simulink model "SERIAL_TRANSMIT_LCD"  (R2021b)
settings: Solver=FixedStepAuto  StartTime=0.0  StopTime=inf  RelTol=1e-3  EnableMultiTasking=on
model workspace (MAT data in the model file):
  x = 1
libraries: arduinolib x2, dspstat3 x2, simulink x1, LCDlib x1
settings Model: ExtModeTrigDuration=2  Creator=kisho  LastModifiedBy=kisho
settings OptimizationCC: EnhancedBackFolding=on  PassReuseOutputArgsAs=Individual arguments  ZeroExternalMemoryAtStartup=off  ZeroInternalMemoryAtStartup=off  MaxStackSize=64  OptimizeBlockOrder=speed  DifferentSizesBufferReuse=on  OptimizationCustomize=off  EfficientTunableParamExpr=on
settings DebuggingCC: ParameterTunabilityLossMsg=error
settings HardwareCC: ProdBitPerInt=16  ProdBitPerPointer=16  ProdBitPerSizeT=16  ProdBitPerPtrDiffT=16  ProdLargestAtomicFloat=None  ProdWordSize=8  ProdHWDeviceType=Atmel->AVR
settings SFSimCC: MATLABDynamicMemAlloc=off
settings RTWCC: Description=Embedded Coder  SystemTargetFile=ert.tlc  HardwareBoard=Arduino Mega 2560  TemplateMakefile=ert_default_tmf  Toolchain=Arduino AVR  BuildConfiguration=Faster Runs
settings CodeAppCC: ForceParamTrailComments=on  IgnoreCustomStorageClasses=off  OperatorAnnotations=on  SimulinkDataObjDesc=on  SFDataObjDesc=on  InsertBlockDesc=on
settings ERTTargetCC: SupportContinuousTime=on  SupportVariableSizeSignals=on  ExtModeTransport=3  ExtModeStaticAlloc=on  ExtModeStaticAllocSize=2048  ExtModeMexFile=ext_xcp  ExtModeIntrfLevel=Level2 - Open

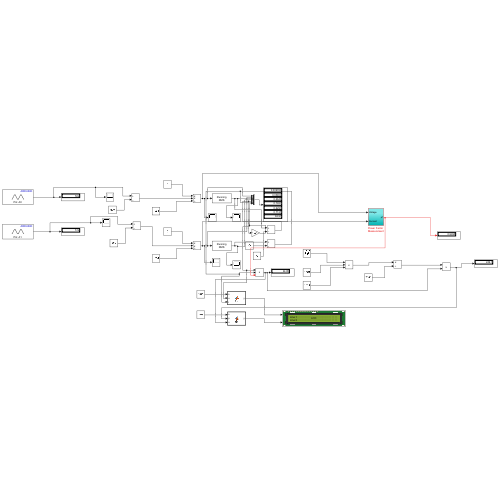
[thumbnail: Simulink's stored preview of the top-level diagram]
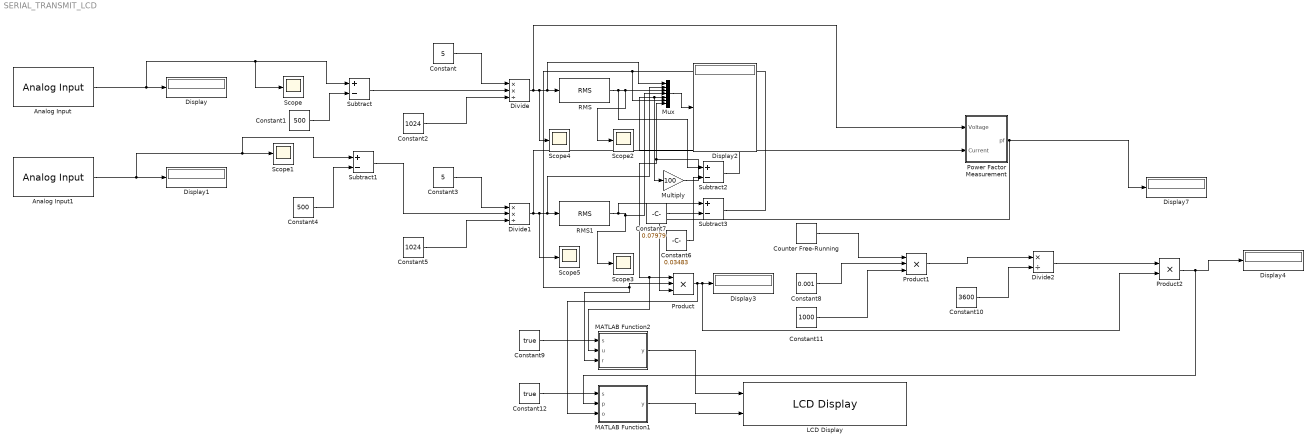
== system SERIAL_TRANSMIT_LCD ==
  Analog Input : arduinolib/Analog Input  pinNumber=0  ReadResultsOnly=off  ConversionTriggerSource=Software  ExternalTriggerType=uint32( 0 )  OutputDataType=uint16  EnableConversionCompleteNotify=off  EnableOuputStatus=off  SampleTime=0.001  blockPlatform=arduino
  Analog Input1 : arduinolib/Analog Input  pinNumber=1  ReadResultsOnly=off  ConversionTriggerSource=Software  ExternalTriggerType=uint32( 0 )  OutputDataType=uint16  EnableConversionCompleteNotify=off  EnableOuputStatus=off  SampleTime=0.001  blockPlatform=arduino
  Constant : Constant  Value=5
  Constant1 : Constant  Value=500
  Constant10 : Constant  Value=3600
  Constant11 : Constant  Value=1000
  Constant12 : Constant  Value=true  OutDataTypeStr=boolean
  Constant2 : Constant  Value=1024
  Constant3 : Constant  Value=5
  Constant4 : Constant  Value=500
  Constant5 : Constant  Value=1024
  Constant6 : Constant  Value=0.03483
  Constant7 : Constant  Value=0.07979
  Constant8 : Constant  Value=0.001
  Constant9 : Constant  Value=true  OutDataTypeStr=boolean
  Counter Free-Running : simulink/Sources/Counter Free-Running  NumBits=32  tsamp=0.001
  Display{,1..4,7} (6 alike) : Display
  Divide : Product  Inputs=**/
  Divide1 : Product  Inputs=**/
  Divide2 : Product  Inputs=*/
  LCD Display : LCDlib/LCD Display  pins=[50, 3, 4, 51, 5, 48]
      settings: SourceProductName=LCD Library
  MATLAB Function1 : MATLAB Function  TreatAsAtomicUnit=on
  MATLAB Function2 : MATLAB Function  TreatAsAtomicUnit=on
  Multiply : Gain  Gain=100
  Mux : Mux  Inputs=7
  Power Factor Measurement : Subsystem
  Product : Product  Inputs=3  OutDataTypeStr=double
  Product1 : Product  Inputs=3
  Product2 : Product
  RMS : dspstat3/RMS  run=on  directionMode=Each column  dimension=1  InputProcessing=Columns as channels (frame based)  reset_popup=None
  RMS1 : dspstat3/RMS  run=on  directionMode=Each column  dimension=1  InputProcessing=Columns as channels (frame based)  reset_popup=None
  Scope{,1..5} (6 alike) : Scope
  Subtract{,1..3} (4 alike) : Sum  Inputs=+-
  wires:
  Constant/1 -> Divide/1
  Constant2/1 -> Divide/3
  RMS/1 -> Mux/3, Scope2/1, Subtract2/1
  Constant3/1 -> Divide1/1
  Analog Input1/1 -> Subtract1/1, Scope1/1, Display1/1
  Constant5/1 -> Divide1/3
  RMS1/1 -> Subtract3/1, Scope3/1, Mux/4
  Analog Input/1 -> Subtract/1, Scope/1, Display/1
  Mux/1 -> Display2/1
  Subtract/1 -> Divide/2
  Constant1/1 -> Subtract/2
  Subtract1/1 -> Divide1/2
  Constant4/1 -> Subtract1/2
  Subtract2/1 -> Multiply/1, Mux/5
  Constant6/1 -> Subtract2/2
  Constant7/1 -> Subtract3/2
  Counter Free-Running/1 -> Product1/1
  Divide2/1 -> Product2/1
  Constant8/1 -> Product1/2
  Constant10/1 -> Divide2/2
  Product1/1 -> Divide2/1
  Product/1 -> MATLAB Function1/3(o), Product2/2, Display3/1
  Constant11/1 -> Product1/3
  Subtract3/1 -> MATLAB Function2/3(r), Product/2, Mux/6
  Multiply/1 -> Mux/7, MATLAB Function2/2(u), Product/1
  Divide/1 -> Power Factor Measurement/1(Voltage), Scope4/1, Mux/1, RMS/1
  Divide1/1 -> RMS1/1, Mux/2, Scope5/1, Power Factor Measurement/2(Current)
  Power Factor Measurement/1(pf) -> Display7/1, Product/3
  Constant9/1 -> MATLAB Function2/1(s)
  Constant12/1 -> MATLAB Function1/1(s)
  MATLAB Function1/1(y) -> LCD Display/2
  MATLAB Function2/1(y) -> LCD Display/1
  Product2/1 -> MATLAB Function1/2(p), Display4/1

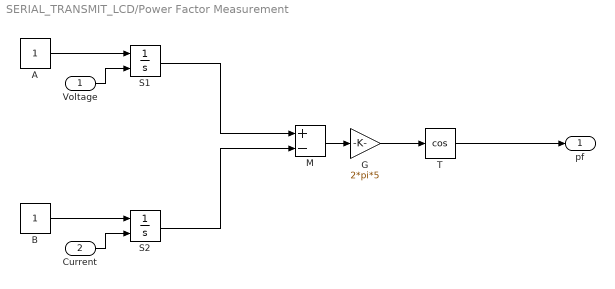
== system SERIAL_TRANSMIT_LCD/Power Factor Measurement ==
  Voltage : Inport
  Current : Inport  Port=2
  A : Constant
  B : Constant
  G : Gain  Gain=2*pi*5
  M : Sum  Inputs=+-
  S1 : Integrator  ExternalReset=falling
  S2 : Integrator  ExternalReset=falling
  T : Trigonometry  Operator=cos
  pf : Outport
  wires:
  A/1 -> S1/1
  B/1 -> S2/1
  S1/1 -> M/1
  S2/1 -> M/2
  Voltage/1 -> S1/2
  Current/1 -> S2/2
  M/1 -> G/1
  G/1 -> T/1
  T/1 -> pf/1

== matlab function SERIAL_TRANSMIT_LCD/MATLAB Function1 ==
  data: s input; p input; y output; o input
function y = fcn(s, p,o)

% Copyright 2008-2019 The MathWorks, Inc.

% s == true  --> energy and power
% u: input numerica data

y           = uint8(zeros([1 16]));

%% first digit
v           = fix(p);
a           = abs(v);
g=fix(o);
k=abs(g);


if a>=0 && a<100
    y(3)    = uint8(48);
    b       = a;
    
elseif a>=100 && a<200
    y(3)    = uint8(49);
    b       = a-100;
    
elseif a>=200 && a<300
    y(3)    = uint8(50);
    b       = a-200;
    
elseif a>=300 && a<400
    y(3)    = uint8(51);
    b       = a-300;
    
elseif a>=400 && a<500
    y(3)    = uint8(52);
    b       = a-400;
    
elseif a>=500 && a<600
    y(3)    = uint8(53);
    b       = a-500;
    
elseif a>=600 && a<700
    y(3)    = uint8(54);
    b       = a-600;
    
elseif a>=700 && a<800
    y(3)    = uint8(55);
    b       = a-700;
    
elseif a>=800 && a<900
    y(3)    = uint8(56);
    b       = a-800;
    
elseif a>=900 && a<1000
    y(3)    = uint8(57);
    b       = a-900;
    
else
    y(3)    = uint8(57);
    b       = 9;
end


if b>=0 && b<10
    y(4)    = uint8(48);
    c       = b;
    
elseif b>=10 && b<20
    y(4)    = uint8(49);
    c       = b-10;
    
elseif b>=20 && b<30
    y(4)    = uint8(50);
    c       = b-20;
    
elseif b>=30 && b<40
    y(4)    = uint8(51);
    c       = b-30;
    
elseif b>=40 && b<50
    y(4)    = uint8(52);
    c       = b-40;
    
elseif b>=50 && b<60
    y(4)    = uint8(53);
    c       = b-50;
    
elseif b>=60 && b<70
    y(4)    = uint8(54);
    c       = a-60;
    
elseif b>=70 && b<80
    y(4)    = uint8(55);
    c       = b-70;
    
elseif b>=80 && b<90
    y(4)    = uint8(56);
    c       = b-80;
    
elseif b>=90 && b<100
    y(4)    = uint8(57);
    c       = a-90;
    
else
    y(4)    = uint8(57);
    c       = 9;
end
if k>=0 && k<10
    y(10)    = uint8(48);
    m       = k;
    
elseif k>=10 && k<20
    y(10)    = uint8(49);
    m       = k-10;
    
elseif k>=20 && k<30
    y(10)    = uint8(50);
    m       = k-20;
    
elseif k>=30 && k<40
    y(10)    = uint8(51);
    m       = k-30;
    
elseif k>=40 && k<50
    y(10)    = uint8(52);
    m       = k-40;
    
elseif k>=50 && k<60
    y(10)    = uint8(53);
    m       = k-50;
    
elseif k>=60 && k<70
    y(10)    = uint8(54);
    m       = k-60;
    
elseif k>=70 && k<80
    y(10)    = uint8(55);
    m       = k-70;
    
elseif k>=80 && k<90
    y(10)    = uint8(56);
    m       = k-80;
    
elseif k>=90 && k<100
    y(10)    = uint8(57);
    m       = k-90;
    
else
    y(10)    = uint8(57);
    m       = 9;
end
%% third digit
y(5)        = determineNumber(c);
y(11)=determineNumber(m);

%% energy and power

if s
    y(1:2)      = uint8([69 58]);
    y(6:7) = uint8([32]);
    y(8:9) = uint8([80 58]);
else
    y(1:6)      = uint8([104   117   109   105    58    32]);
    y([12 13])  = uint8([32 37]);
end

end



%% local helper function

function d = determineNumber(n)

    switch n
        case 0
            d = uint8(48);
        case 1
            d = uint8(49);
        case 2
            d = uint8(50);
        case 3
            d = uint8(51);
        case 4
            d = uint8(52);
        case 5
            d = uint8(53);
        case 6
            d = uint8(54);
        case 7
            d = uint8(55);
        case 8
            d = uint8(56);
        case 9
            d = uint8(57);    
        otherwise
            d = uint8(57);
    end

end

== matlab function SERIAL_TRANSMIT_LCD/MATLAB Function2 ==
  data: s input; u input; y output; r input
function y = fcn(s, u,r)

% Copyright 2008-2019 The MathWorks, Inc.

% s == true  --> voltage and current
% u: input numerica data

y           = uint8(zeros([1 16]));

%% first digit
v           = fix(u);
a           = abs(v);
t           = r;
l           = t*100;

if a>=0 && a<10
    y(3)    = uint8(48);
    b       = a;
    
elseif a>=10 && a<20
    y(3)    = uint8(49);
    b       = a-10;
    
elseif a>=20 && a<30
    y(3)    = uint8(50);
    b       = a-20;
    
elseif a>=30 && a<40
    y(3)    = uint8(51);
    b       = a-30;
    
elseif a>=40 && a<50
    y(3)    = uint8(52);
    b       = a-40;
    
elseif a>=50 && a<60
    y(3)    = uint8(53);
    b       = a-50;
    
elseif a>=60 && a<70
    y(3)    = uint8(54);
    b       = a-60;
    
elseif a>=70 && a<80
    y(3)    = uint8(55);
    b       = a-70;
    
elseif a>=80 && a<90
    y(3)    = uint8(56);
    b       = a-80;
    
elseif a>=90 && a<100
    y(3)    = uint8(57);
    b       = a-90;
    
else
    y(3)    = uint8(57);
    b       = 9;
end

if l>=0 && l<10
    y(12)    = uint8(48);
    c       = l;
    
elseif l>=10 && l<20
    y(12)    = uint8(49);
    c       = l-10;
    
elseif l>=20 && l<30
    y(12)    = uint8(50);
    c       = l-20;
    
elseif l>=30 && l<40
    y(12)    = uint8(51);
    c       = l-30;
    
elseif l>=40 && l<50
    y(12)    = uint8(52);
    c       = l-40;
    
elseif l>=50 && l<60
    y(12)    = uint8(53);
    c       = l-50;
    
elseif l>=60 && l<70
    y(12)    = uint8(54);
    c       = l-60;
    
elseif l>=70 && l<80
    y(12)    = uint8(55);
    c       = l-70;
    
elseif l>=80 && l<90
    y(12)    = uint8(56);
    c       = l-80;
    
elseif l>=90 && l<100
    y(12)    = uint8(57);
    c       = l-90;
    
else
    y(12)    = uint8(57);
    c       = 9;
end


%% second digit
y(4)        = determineNumber(b);
y(13)        = determineNumber(c);

%% fractional part
f           = fix((u-v)*10);

y(5)       = uint8(46);
y(6)       = determineNumber(f);

y(11)       = uint8(46);
y(10)=uint8(48);
y(7)=uint8(32);


%% voltage and current

if s
    y(1:2)      = uint8([86 58]);
    y(8:9)  = uint8([73 58]);
else
    y(1:6)      = uint8([104   117   109   105    58    32]);
    y([12 13])  = uint8([32 37]);
end

end



%% local helper function

function d = determineNumber(n)

    switch n
        case 0
            d = uint8(48);
        case 1
            d = uint8(49);
        case 2
            d = uint8(50);
        case 3
            d = uint8(51);
        case 4
            d = uint8(52);
        case 5
            d = uint8(53);
        case 6
            d = uint8(54);
        case 7
            d = uint8(55);
        case 8
            d = uint8(56);
        case 9
            d = uint8(57);    
        otherwise
            d = uint8(57);
    end

end
